simulink model "New_tread_carcass_thermal_model"  (R2024b)
settings: Solver=VariableStepAuto  StartTime=0  StopTime=2105  FixedStep=0.01  MaxStep=0.5  RelTol=1e-4
undefined symbols (not defined in the file): a_cp, cs, data, Fx, Fy, Fz, h_tt, M_tread, p1, p2, p3, Rl, S_tread, SA, SL, T_amb, T_track, TSTC, Vx
settings Model: Creator=Utente  LastModifiedBy=Utente

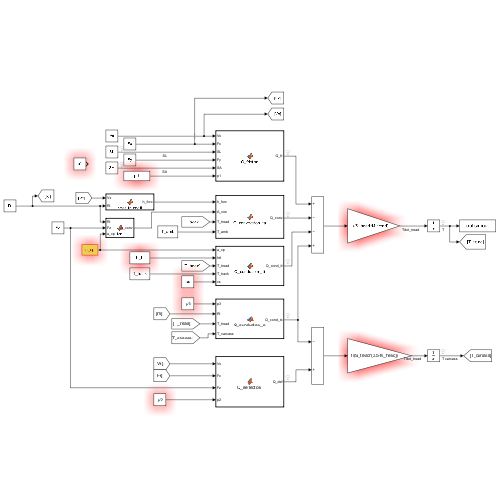
[thumbnail: Simulink's stored preview of the top-level diagram]
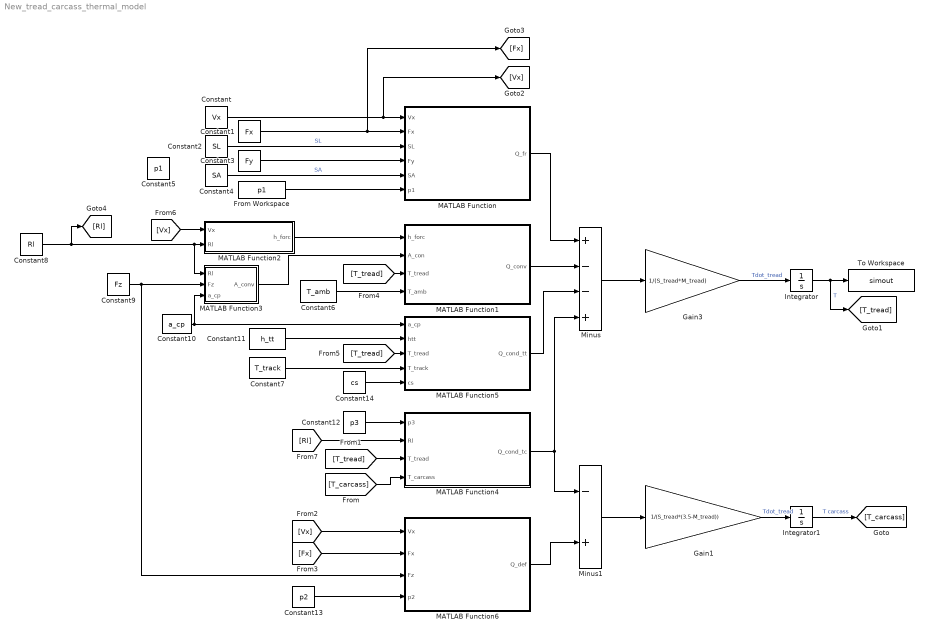
== system New_tread_carcass_thermal_model ==
  Constant : Constant  Value=Vx
  Constant1 : Constant  Value=Fx
  Constant10 : Constant  Value=a_cp
  Constant11 : Constant  Value=h_tt
  Constant12 : Constant  Value=p3
  Constant13 : Constant  Value=p2
  Constant14 : Constant  Value=cs
  Constant2 : Constant  Value=SL
  Constant3 : Constant  Value=Fy
  Constant4 : Constant  Value=SA
  Constant5 : Constant  Value=p1
  Constant6 : Constant  Value=T_amb
  Constant7 : Constant  Value=T_track
  Constant8 : Constant  Value=Rl
  Constant9 : Constant  Value=Fz
  From Workspace : FromWorkspace  VariableName=p1
  Gain1 : Gain  Gain=1/(S_tread*(3.5-M_tread))
  Gain3 : Gain  Gain=1/(S_tread*M_tread)
  Integrator : Integrator  InitialCondition=data.TSTC(1)
  Integrator1 : Integrator  InitialCondition=TSTC(1)
  MATLAB Function : MATLAB Function  TreatAsAtomicUnit=on
  MATLAB Function1 : MATLAB Function  TreatAsAtomicUnit=on
  MATLAB Function2 : MATLAB Function  TreatAsAtomicUnit=on
  MATLAB Function3 : MATLAB Function  TreatAsAtomicUnit=on
  MATLAB Function4 : MATLAB Function  TreatAsAtomicUnit=on
  MATLAB Function5 : MATLAB Function  TreatAsAtomicUnit=on
  MATLAB Function6 : MATLAB Function  TreatAsAtomicUnit=on
  Minus : Sum  Inputs=+--+
  Minus1 : Sum  Inputs=-+
  To Workspace : ToWorkspace  VariableName=simout  SaveFormat=Timeseries  SampleTime=-1
  wires:
  Gain3/1 -> Integrator/1  "Tdot_tread"
  Integrator/1 -> [T_tread], To Workspace/1  "T"
  Gain1/1 -> Integrator1/1  "Tdot_tread"
  MATLAB Function2/1(h_forc) -> MATLAB Function1/1(h_forc)
  MATLAB Function3/1(A_conv) -> MATLAB Function1/2(A_con)
  Minus/1 -> Gain3/1
  MATLAB Function/1(Q_fr) -> Minus/1
  MATLAB Function1/1(Q_conv) -> Minus/2
  MATLAB Function5/1(Q_cond_tt) -> Minus/3
  MATLAB Function4/1(Q_cond_tc) -> Minus/4, Minus1/1
  MATLAB Function6/1(Q_def) -> Minus1/2
  Minus1/1 -> Gain1/1
  Integrator1/1 -> [T_carcass]  "T carcass"
  [T_carcass] -> MATLAB Function4/4(T_carcass)
  [T_tread] -> MATLAB Function4/3(T_tread)
  Constant/1 -> [Vx], MATLAB Function/1(Vx)
  Constant1/1 -> [Fx], MATLAB Function/2(Fx)
  Constant2/1 -> MATLAB Function/3(SL)  "SL"
  Constant3/1 -> MATLAB Function/4(Fy)
  Constant4/1 -> MATLAB Function/5(SA)  "SA"
  From Workspace/1 -> MATLAB Function/6(p1)
  [Vx] -> MATLAB Function6/1(Vx)
  [Fx] -> MATLAB Function6/2(Fx)
  [T_tread] -> MATLAB Function1/3(T_tread)
  Constant6/1 -> MATLAB Function1/4(T_amb)
  [T_tread] -> MATLAB Function5/3(T_tread)
  Constant8/1 -> [Rl], MATLAB Function3/1(Rl), MATLAB Function2/2(Rl)
  [Vx] -> MATLAB Function2/1(Vx)
  Constant10/1 -> MATLAB Function3/3(a_cp), MATLAB Function5/1(a_cp)
  Constant9/1 -> MATLAB Function6/3(Fz), MATLAB Function3/2(Fz)
  Constant7/1 -> MATLAB Function5/4(T_track)
  Constant11/1 -> MATLAB Function5/2(htt)
  [Rl] -> MATLAB Function4/2(Rl)
  Constant12/1 -> MATLAB Function4/1(p3)
  Constant13/1 -> MATLAB Function6/4(p2)
  Constant14/1 -> MATLAB Function5/5(cs)

== matlab function New_tread_carcass_thermal_model/MATLAB Function1 ==
  data: h_forc input; Q_conv output; A_con input; T_tread input; T_amb input
function Q_conv = Q_convectrion_ta(h_forc, A_con, T_tread, T_amb)

Q_conv = h_forc*A_conv*(T_tread - T_Amb)
end

== matlab function New_tread_carcass_thermal_model/MATLAB Function ==
  data: Vx input; Q_fr output; Fx input; SL input; Fy input; SA input; p1 input
function Q_fr = Q_friction(Vx, Fx, SL, Fy, SA, p1)


Q_fr = p1*Vx*(Fx*SL + Fy*SA)
end

== matlab function New_tread_carcass_thermal_model/MATLAB Function2 ==
  data: Vx input; Rl input; h_forc output
function h_forc = heat_tr_coeff(Vx,Rl)
W = 0.1905;
D = 2*Rl;
K_air = 28.08;
nu_air = 0.3685;


L = 1/(1/W + 1/D);

h_forc = K_air/L *(0.0239*(Vx*L/nu_air)^0.805);

== matlab function New_tread_carcass_thermal_model/MATLAB Function3 ==
  data: Rl input; A_conv output; Fz input; a_cp input
function A_conv = fcn(Rl, Fz, a_cp)
W = 0.1905;
cl = a_cp * Fz^0.7; % da ottimizzatore

Atot = pi*2*Rl * W;
A_conv = Atot - W*cl;
end

== matlab function New_tread_carcass_thermal_model/MATLAB Function4 ==
  data: p3 input; Rl input; T_tread input; Q_cond_tc output; T_carcass input
function  Q_cond_tc = Q_conduction_tc(p3,Rl,  T_tread, T_carcass)
W = 0.1905;
A_tot = pi*W*2*Rl;
Q_cond_tc = p3*A_tot*(T_tread - T_carcass);
end

== matlab function New_tread_carcass_thermal_model/MATLAB Function5 ==
  data: a_cp input; htt input; Q_cond_tt output; T_tread input; T_track input; cs input
function  Q_cond_tt = Q_conduction_tt(a_cp, htt,  T_tread, T_track,cs)
W = 0.1905;
cl = a_cp * Fz^0.7;
A_cp = cl*cs*W;
Q_cond_tt = htt*A_cp*(T_tread - T_track);
end

== matlab function New_tread_carcass_thermal_model/MATLAB Function6 ==
  data: Vx input; Q_def output; Fx input; Fz input; p2 input
function Q_def = Q_deflection(Vx, Fx, Fz, p2)


Q_def = p2*Vx*(Vx*Fx^2/Fz);
end
